simulink model "mpc_con"  (R2019b)
settings: Solver=VariableStepAuto  StartTime=0.0  StopTime=time_end  RelTol=1e-3
values from neighbouring files (symbols this model uses):
  h_01 = 10.17    [script_mpc_con.m]
  h_02 = 10.53    [script_mpc_con.m]
  Td = 0.5    [script_mpc_con.m]
  u_max = repmat(u_max,Nc,1)    [script_mpc_con.m]
  u_min = repmat(u_min,Nc,1)    [script_mpc_con.m]
  ue = [ue1; ue2]    [script_mpc_con.m]
  x_max = repmat(x_max,Np,1)    [script_mpc_con.m]
  x_min = repmat(x_min,Np,1)    [script_mpc_con.m]
  xe = [xe1; xe2]    [script_mpc_con.m]
undefined symbols (not defined in the file or in its folder): A, B, C, Fx, Fy, Gx, Gy
settings Model: Creator=NicSch02  LastModifiedBy=NicSch02

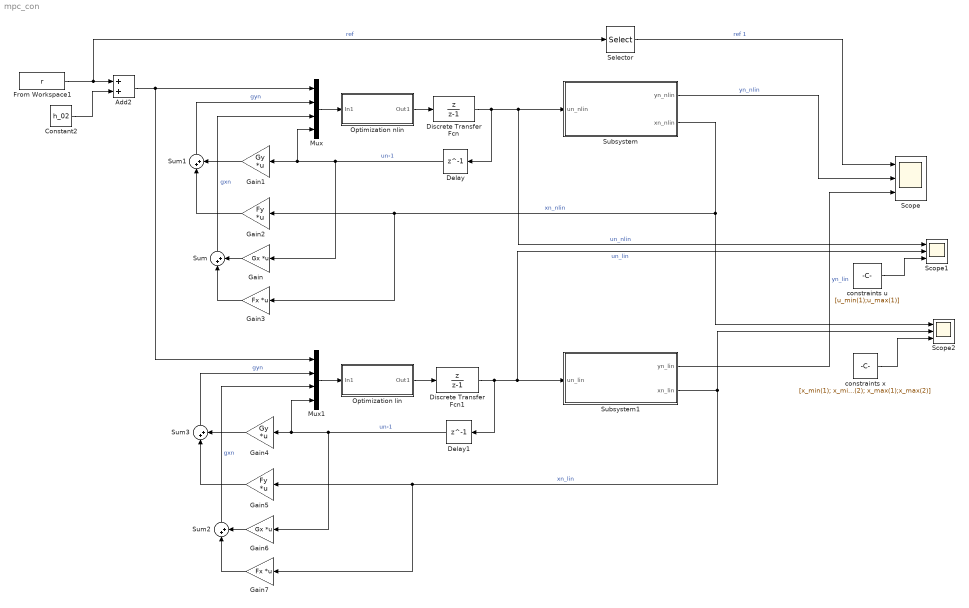
== system mpc_con ==
  Add2 : Sum
  Constant2 : Constant  Value=h_02
  Delay : Delay  DelayLength=1  InitialCondition=[0;0]  SampleTime=Td
  Delay1 : Delay  DelayLength=1  InitialCondition=[0;0]  SampleTime=Td
  Discrete Transfer Fcn : DiscreteTransferFcn  Numerator=[1 0]  Denominator=[1 -1]  InitialStates=[0;0]  SampleTime=Td
  Discrete Transfer Fcn1 : DiscreteTransferFcn  Numerator=[1 0]  Denominator=[1 -1]  InitialStates=[0;0]  SampleTime=Td
  From Workspace1 : FromWorkspace  VariableName=r  SampleTime=0
  Gain : Gain  Gain=Gx  Multiplication=Matrix(K*u)
  Gain1 : Gain  Gain=Gy  Multiplication=Matrix(K*u)
  Gain2 : Gain  Gain=Fy  Multiplication=Matrix(K*u)
  Gain3 : Gain  Gain=Fx  Multiplication=Matrix(K*u)
  Gain4 : Gain  Gain=Gy  Multiplication=Matrix(K*u)
  Gain5 : Gain  Gain=Fy  Multiplication=Matrix(K*u)
  Gain6 : Gain  Gain=Gx  Multiplication=Matrix(K*u)
  Gain7 : Gain  Gain=Fx  Multiplication=Matrix(K*u)
  Mux : Mux
  Mux1 : Mux
  Optimization lin : Subsystem  TreatAsAtomicUnit=on  SystemSampleTime=Td
  Optimization nlin : Subsystem  TreatAsAtomicUnit=on  SystemSampleTime=Td
  Scope : Scope  NumInputPorts=3
  Scope1 : Scope  NumInputPorts=3
  Scope2 : Scope  NumInputPorts=3
  Selector : Selector  InputPortWidth=Np  IndexOptions=Index vector (dialog)  Indices=[1]  OutputSizes=1
  Subsystem : Subsystem
  Subsystem1 : Subsystem
  Sum{,1..3} (4 alike) : Sum  Inputs=|++
  constraints u : Constant  Value=[u_min(1);u_max(1)]
  constraints x : Constant  Value=[x_min(1); x_min(2); x_max(1);x_max(2)]
  wires:
  Discrete Transfer Fcn/1 -> Scope1/1, Subsystem/1(un_nlin), Delay/1  "un_nlin"
  Delay/1 -> Gain/1, Mux/4, Gain1/1  "un-1"
  Gain1/1 -> Sum1/2
  Sum1/1 -> Mux/2  "gyn"
  Gain2/1 -> Sum1/1
  Subsystem/1(yn_nlin) -> Scope/2  "yn_nlin"
  Discrete Transfer Fcn1/1 -> Scope1/2, Subsystem1/1(un_lin), Delay1/1  "un_lin"
  Gain4/1 -> Sum3/2
  Gain5/1 -> Sum3/1
  Subsystem1/1(yn_lin) -> Scope/3  "yn_lin"
  Subsystem/2(xn_nlin) -> Gain3/1, Gain2/1, Scope2/1  "xn_nlin"
  Subsystem1/2(xn_lin) -> Gain7/1, Gain5/1, Scope2/2  "xn_lin"
  Selector/1 -> Scope/1  "ref 1"
  Mux/1 -> Optimization nlin/1(In1)
  Sum3/1 -> Mux1/2  "gyn"
  Mux1/1 -> Optimization lin/1(In1)
  Optimization nlin/1(Out1) -> Discrete Transfer Fcn/1
  Optimization lin/1(Out1) -> Discrete Transfer Fcn1/1
  Gain/1 -> Sum/2
  Gain3/1 -> Sum/1
  Sum/1 -> Mux/3  "gxn"
  Gain6/1 -> Sum2/2
  Delay1/1 -> Gain6/1, Mux1/4, Gain4/1  "un-1"
  Sum2/1 -> Mux1/3  "gxn"
  Gain7/1 -> Sum2/1
  Constant2/1 -> Add2/2
  From Workspace1/1 -> Selector/1, Add2/1  "ref"
  Add2/1 -> Mux1/1, Mux/1
  constraints x/1 -> Scope2/3
  constraints u/1 -> Scope1/3

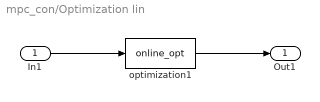
== system mpc_con/Optimization lin ==
  In1 : Inport
  optimization1 : MATLABFcn  MATLABFcn=online_opt
  Out1 : Outport
  wires:
  In1/1 -> optimization1/1
  optimization1/1 -> Out1/1

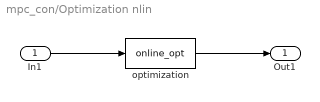
== system mpc_con/Optimization nlin ==
  In1 : Inport
  optimization : MATLABFcn  MATLABFcn=online_opt
  Out1 : Outport
  wires:
  In1/1 -> optimization/1
  optimization/1 -> Out1/1

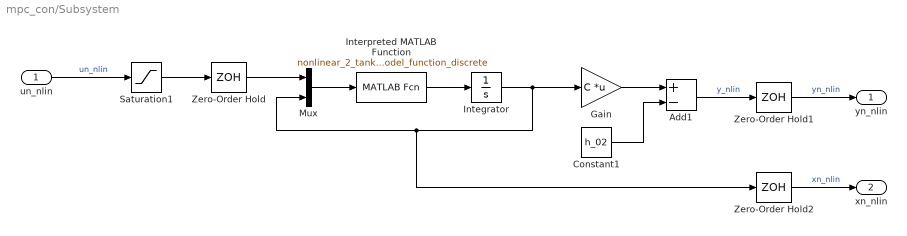
== system mpc_con/Subsystem ==
  un_nlin : Inport
  Add1 : Sum  Inputs=+-
  Constant1 : Constant  Value=h_02
  Gain : Gain  Gain=C  Multiplication=Matrix(K*u)
  Integrator : Integrator  InitialCondition=[h_01;h_02]
  Interpreted MATLAB Function : MATLABFcn  MATLABFcn=nonlinear_2_tank_model_function_discrete
  Mux : Mux  Inputs=2
  Saturation1 : Saturate  UpperLimit=u_max(1)  LowerLimit=u_min(1)
  Zero-Order Hold : ZeroOrderHold  SampleTime=Td
  Zero-Order Hold1 : ZeroOrderHold  SampleTime=Td
  Zero-Order Hold2 : ZeroOrderHold  SampleTime=Td
  yn_nlin : Outport
  xn_nlin : Outport  Port=2
  wires:
  Integrator/1 -> Zero-Order Hold2/1, Mux/2, Gain/1
  Constant1/1 -> Add1/2
  Interpreted MATLAB Function/1 -> Integrator/1
  Gain/1 -> Add1/1
  Mux/1 -> Interpreted MATLAB Function/1
  un_nlin/1 -> Saturation1/1  "un_nlin"
  Zero-Order Hold/1 -> Mux/1
  Add1/1 -> Zero-Order Hold1/1  "y_nlin"
  Zero-Order Hold1/1 -> yn_nlin/1  "yn_nlin"
  Saturation1/1 -> Zero-Order Hold/1
  Zero-Order Hold2/1 -> xn_nlin/1  "xn_nlin"

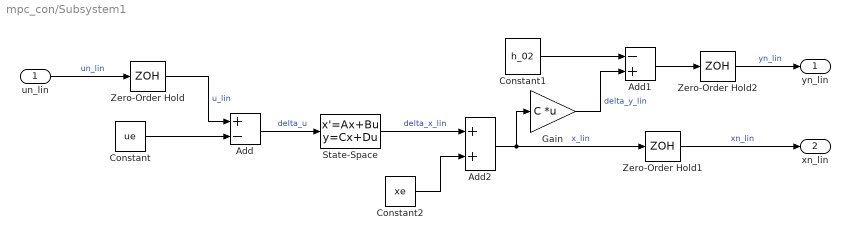
== system mpc_con/Subsystem1 ==
  un_lin : Inport
  Add : Sum  Inputs=+-
  Add1 : Sum  Inputs=-+
  Add2 : Sum
  Constant : Constant  Value=ue
  Constant1 : Constant  Value=h_02
  Constant2 : Constant  Value=xe
  Gain : Gain  Gain=C  Multiplication=Matrix(K*u)
  State-Space : StateSpace  A=A  B=B  C=[[1,0];[0,1]]  D=[[0,0];[0,0]]  InitialCondition=[h_01;h_02] - xe
  Zero-Order Hold : ZeroOrderHold  SampleTime=Td
  Zero-Order Hold1 : ZeroOrderHold  SampleTime=Td
  Zero-Order Hold2 : ZeroOrderHold  SampleTime=Td
  yn_lin : Outport
  xn_lin : Outport  Port=2
  wires:
  Constant/1 -> Add/2
  Add/1 -> State-Space/1  "delta_u"
  Constant2/1 -> Add2/2
  State-Space/1 -> Add2/1  "delta_x_lin"
  un_lin/1 -> Zero-Order Hold/1  "un_lin"
  Zero-Order Hold/1 -> Add/1  "u_lin"
  Add2/1 -> Zero-Order Hold1/1, Gain/1  "x_lin"
  Zero-Order Hold1/1 -> xn_lin/1  "xn_lin"
  Zero-Order Hold2/1 -> yn_lin/1  "yn_lin"
  Add1/1 -> Zero-Order Hold2/1
  Constant1/1 -> Add1/1
  Gain/1 -> Add1/2  "delta_y_lin"
